simulink model "sol6_step_without_windup"  (R2021b)
settings: Solver=VariableStepAuto  StartTime=0.0  StopTime=2  RelTol=1e-3
PreLoadFcn:
  | initModelData
  | trajectoryData
  | controlPID
StartFcn:
  | controlPID
values from neighbouring files (symbols this model uses):
  B = Bm+(Kb*Km/R)    (= 0.0149065789474)    [MyData_for_1_and_2.m]    (also in MyData_for_3_4_and_5.m; MyData_for_5_and_6.m)
  Jm = 5.5e-4    (= 0.00055)    [MyData_for_1_and_2.m]    (also in MyData_for_3_4_and_5.m; MyData_for_5_and_6.m)
  Kd = (R/Km)*((2*Jm*w*zeta)-B)    (= 0.369819047619)    [MyData_for_1_and_2.m]    (also in MyData_for_3_4_and_5.m = 0.2902; MyData_for_5_and_6.m = 0.0513428571429)
  Km = 0.105    [MyData_for_1_and_2.m]    (also in MyData_for_3_4_and_5.m; MyData_for_5_and_6.m)
  Kp = (R/Km)*(Jm*(w^2))    (= 14.3314285714)    [MyData_for_1_and_2.m]    (also in MyData_for_3_4_and_5.m = 9.95238095238; MyData_for_5_and_6.m = 1.59238095238)
  R = 0.76    [MyData_for_1_and_2.m]    (also in MyData_for_3_4_and_5.m; MyData_for_5_and_6.m)
  r = 156    [MyData_for_1_and_2.m]    (also in MyData_for_3_4_and_5.m; MyData_for_5_and_6.m)
undefined symbols (not defined in the file or in its folder): Ki
settings Model: Creator=esdan  LastModifiedBy=munir
settings SolverCC: AlgebraicLoopSolver=TrustRegion
settings DebuggingCC: SFMachineParentedDataDiag=warning

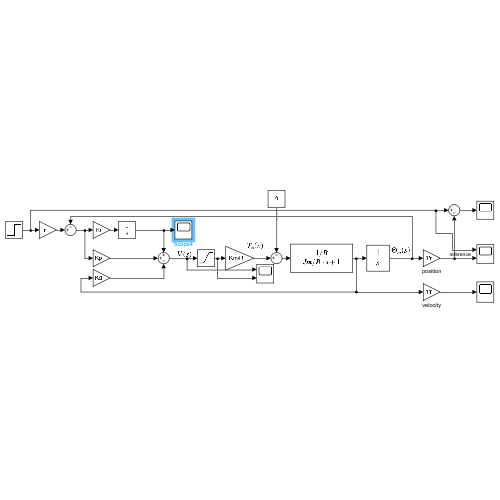
[thumbnail: Simulink's stored preview of the top-level diagram]
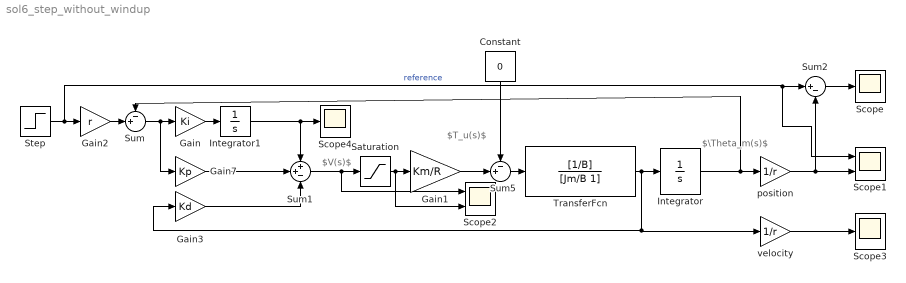
== system sol6_step_without_windup ==
  note: $\Theta_m(s)$
  note: $V(s)$
  note: $T_u(s)$
  Constant : Constant  Value=0
  Gain : Gain  Gain=Ki
  Gain1 : Gain  Gain=Km/R
  Gain2 : Gain  Gain=r
  Gain3 : Gain  Gain=Kd
  Gain7 : Gain  Gain=Kp
  Integrator : Integrator
  Integrator1 : Integrator
  Saturation : Saturate  UpperLimit=35  LowerLimit=-35
  Scope : Scope
  Scope1 : Scope  NumInputPorts=2
  Scope2 : Scope  NumInputPorts=2
  Scope3 : Scope
  Scope4 : Scope
  Step : Step  Time=0.5  After=.5  SampleTime=0
  Sum : Sum  Inputs=-+|
  Sum1 : Sum  Inputs=++-
  Sum2 : Sum  Inputs=|+-
  Sum5 : Sum  Inputs=-+|
  TransferFcn : TransferFcn  Numerator=[1/B]  Denominator=[Jm/B 1]
  position : Gain  Gain=1/r
  velocity : Gain  Gain=1/r
  wires:
  Saturation/1 -> Scope2/2, Gain1/1
  Sum/1 -> Gain7/1, Gain/1
  Sum1/1 -> Scope2/1, Saturation/1
  Gain2/1 -> Sum/2
  Step/1 -> Scope1/1, Sum2/1, Gain2/1  "reference"
  Sum2/1 -> Scope/1
  TransferFcn/1 -> Integrator/1, velocity/1, Gain3/1
  position/1 -> Scope1/2, Sum2/2
  Integrator/1 -> position/1, Sum/1
  Sum5/1 -> TransferFcn/1
  Gain1/1 -> Sum5/2
  Gain3/1 -> Sum1/3
  Gain7/1 -> Sum1/2
  Integrator1/1 -> Sum1/1, Scope4/1
  Gain/1 -> Integrator1/1
  velocity/1 -> Scope3/1
  Constant/1 -> Sum5/1
